simulink subsystem "Out_of_Plane_Model"  (R2025b)
settings: Solver=VariableStepAuto  StartTime=0.0  StopTime=10.0  RelTol=1e-3
undefined symbols (not defined in the file): AeroLiftCff, AeroLongDrgCff, AeroMotoEffctArea, AeroPitchMomentCff, AeroPitchMomentLngth, AeroRltWindAngVect, AeroSideFrcCff, AeroYawMomentCff, aMode, BrkFrntBrkActrBore, BrkFrntBrkActrPrsBpt, BrkFrntBrkPadMeanRadius, BrkFrntBrkTrqTbl, BrkFrntIntrnRadius, BrkFrntKinFricCff, BrkFrntPadNum, BrkFrntShoePinToDrumCntrDst, BrkFrntShoePinToFrcAppDst, BrkFrntShoePinToPadEndAng, BrkFrntShoePinToPadStartAng, BrkFrntStcFricCff, BrkFrntWhlSpdBpt, BrkRearBrkActrBore, BrkRearBrkActrPrsBpt, BrkRearBrkPadMeanRadius, BrkRearBrkTrqTbl, BrkRearIntrnRadius, BrkRearKinFricCff, BrkRearPadNum, BrkRearShoePinToDrumCntrDst, BrkRearShoePinToFrcAppDst, BrkRearShoePinToPadEndAng, BrkRearShoePinToPadStartAng, BrkRearStcFricCff, BrkRearWhlSpdBpt, CpRrVx0, CpRrVy0, CpRrY0, EnvAbsPrs, EnvAirTemp, FrkFrL0, FrmAng0, g, GasCnst, InitFrkLngth, InitMainFrmPitchAng, InitRearArmPitchAng, InitRearCntctPtchLatVel, InitRearCntctPtchLongVel, InitRearCntctPtchZ, InitYawAng, MotoFrmLngth, MotoFrmMass, MotoGrvty, MotoLatOfst, MotoLongOfst, MotoLowrFrntFrkMass, MotoPtchOfst, MotoRearArmLngth, MotoRearArmMass ... (+28)
libraries: sm_lib x309, nesl_utility_internal x158, nesl_utility x7, autolibsharedcoupling x6, vehdynlibtire x6, sharedtransform x4, shared6dof x1, matrix_library x1, vehdynlibeomcommon x1
(part 9 of 10)

== system Out_of_Plane_Model/Chassis, Tires, and Areo/Chassis Body, Suspension, and Steering/Signal routine/Ancillary_sub/Velocities/Sensor/Sensor_FrkLw ==
  PS-Simulink Converter1 : nesl_utility_internal/PS-Simulink Converter  PhysicalDomain=network_engine_domain  SubClassName=ps_output  LeftPortType=input  RightPortType=output  PseudoPeriodic=off  Frequencies=[]  VectorFormat=1-D array  Unit=inherit  AffineConversion=off
  PS-Simulink Converter4 : nesl_utility_internal/PS-Simulink Converter  PhysicalDomain=network_engine_domain  SubClassName=ps_output  LeftPortType=input  RightPortType=output  PseudoPeriodic=off  Frequencies=[]  VectorFormat=1-D array  Unit=inherit  AffineConversion=off
  PS-Simulink Converter5 : nesl_utility_internal/PS-Simulink Converter  PhysicalDomain=network_engine_domain  SubClassName=ps_output  LeftPortType=input  RightPortType=output  PseudoPeriodic=off  Frequencies=[]  VectorFormat=1-D array  Unit=inherit  AffineConversion=off
  Transform Sensor1 : sm_lib/Frames and Transforms/Transform Sensor  MeasurementFrame=NonRotatingFollower  RotationSequence=XYX  SenseAngle=off  SenseAxis=off  SenseQ=off  SenseR=off  SenseRotationSequence=off  SenseOmegaX=off  SenseOmegaY=off  SenseOmegaZ=off  SenseOmega=off  SenseQDot=off  SenseRDot=off  SenseRotationSequenceDot=off  SenseAlphaX=off  SenseAlphaY=off  SenseAlphaZ=off  SenseAlpha=off  SenseQDDot=off  SenseRDDot=off  SenseX=off  SenseY=off  SenseZ=off  SenseXYZ=off  SenseRad=off  SenseAzim=off  SenseDist=off  SenseInc=off  SenseXDot=on  SenseYDot=on  SenseZDot=on  SenseXYZDot=off  SenseRadDot=off  SenseAzimDot=off  SenseDistDot=off  SenseIncDot=off  SenseXDDot=off  SenseYDDot=off  SenseZDDot=off  SenseXYZDDot=off  SenseRadDDot=off  SenseAzimDDot=off  SenseDistDDot=off  SenseIncDDot=off
  World Frame : sm_lib/Frames and Transforms/World Frame
  F : PMIOPort  Side=Left
  Vx_vf : Outport
  Vy_vf : Outport  Port=2
  Vz_vf : Outport  Port=3
  wires:
  PS-Simulink Converter5/1 -> Vy_vf/1
  PS-Simulink Converter4/1 -> Vx_vf/1
  PS-Simulink Converter1/1 -> Vz_vf/1
  connections:
  World Frame/RConn1 -- Transform Sensor1/LConn1
  Transform Sensor1/RConn1 -- F/RConn1
  PS-Simulink Converter5/LConn1 -- Transform Sensor1/RConn3
  PS-Simulink Converter4/LConn1 -- Transform Sensor1/RConn2
  PS-Simulink Converter1/LConn1 -- Transform Sensor1/RConn4

== system Out_of_Plane_Model/Chassis, Tires, and Areo/Chassis Body, Suspension, and Steering/Signal routine/Ancillary_sub/Velocities/Sensor/Sensor_FrkUp ==
  PS-Simulink Converter1 : nesl_utility_internal/PS-Simulink Converter  PhysicalDomain=network_engine_domain  SubClassName=ps_output  LeftPortType=input  RightPortType=output  PseudoPeriodic=off  Frequencies=[]  VectorFormat=1-D array  Unit=inherit  AffineConversion=off
  PS-Simulink Converter4 : nesl_utility_internal/PS-Simulink Converter  PhysicalDomain=network_engine_domain  SubClassName=ps_output  LeftPortType=input  RightPortType=output  PseudoPeriodic=off  Frequencies=[]  VectorFormat=1-D array  Unit=inherit  AffineConversion=off
  PS-Simulink Converter5 : nesl_utility_internal/PS-Simulink Converter  PhysicalDomain=network_engine_domain  SubClassName=ps_output  LeftPortType=input  RightPortType=output  PseudoPeriodic=off  Frequencies=[]  VectorFormat=1-D array  Unit=inherit  AffineConversion=off
  Transform Sensor1 : sm_lib/Frames and Transforms/Transform Sensor  MeasurementFrame=NonRotatingFollower  RotationSequence=XYX  SenseAngle=off  SenseAxis=off  SenseQ=off  SenseR=off  SenseRotationSequence=off  SenseOmegaX=off  SenseOmegaY=off  SenseOmegaZ=off  SenseOmega=off  SenseQDot=off  SenseRDot=off  SenseRotationSequenceDot=off  SenseAlphaX=off  SenseAlphaY=off  SenseAlphaZ=off  SenseAlpha=off  SenseQDDot=off  SenseRDDot=off  SenseX=off  SenseY=off  SenseZ=off  SenseXYZ=off  SenseRad=off  SenseAzim=off  SenseDist=off  SenseInc=off  SenseXDot=on  SenseYDot=on  SenseZDot=on  SenseXYZDot=off  SenseRadDot=off  SenseAzimDot=off  SenseDistDot=off  SenseIncDot=off  SenseXDDot=off  SenseYDDot=off  SenseZDDot=off  SenseXYZDDot=off  SenseRadDDot=off  SenseAzimDDot=off  SenseDistDDot=off  SenseIncDDot=off
  World Frame : sm_lib/Frames and Transforms/World Frame
  F : PMIOPort  Side=Left
  Vx_vf : Outport
  Vy_vf : Outport  Port=2
  Vz_vf : Outport  Port=3
  wires:
  PS-Simulink Converter1/1 -> Vz_vf/1
  PS-Simulink Converter4/1 -> Vx_vf/1
  PS-Simulink Converter5/1 -> Vy_vf/1
  connections:
  PS-Simulink Converter1/LConn1 -- Transform Sensor1/RConn4
  PS-Simulink Converter4/LConn1 -- Transform Sensor1/RConn2
  PS-Simulink Converter5/LConn1 -- Transform Sensor1/RConn3
  Transform Sensor1/RConn1 -- F/RConn1
  World Frame/RConn1 -- Transform Sensor1/LConn1

== system Out_of_Plane_Model/Chassis, Tires, and Areo/Chassis Body, Suspension, and Steering/Signal routine/Ancillary_sub/Velocities/Sensor/Sensor_Frm ==
  PS-Simulink Converter1 : nesl_utility_internal/PS-Simulink Converter  PhysicalDomain=network_engine_domain  SubClassName=ps_output  LeftPortType=input  RightPortType=output  PseudoPeriodic=off  Frequencies=[]  VectorFormat=1-D array  Unit=inherit  AffineConversion=off
  PS-Simulink Converter4 : nesl_utility_internal/PS-Simulink Converter  PhysicalDomain=network_engine_domain  SubClassName=ps_output  LeftPortType=input  RightPortType=output  PseudoPeriodic=off  Frequencies=[]  VectorFormat=1-D array  Unit=inherit  AffineConversion=off
  PS-Simulink Converter5 : nesl_utility_internal/PS-Simulink Converter  PhysicalDomain=network_engine_domain  SubClassName=ps_output  LeftPortType=input  RightPortType=output  PseudoPeriodic=off  Frequencies=[]  VectorFormat=1-D array  Unit=inherit  AffineConversion=off
  Transform Sensor1 : sm_lib/Frames and Transforms/Transform Sensor  MeasurementFrame=NonRotatingFollower  RotationSequence=XYX  SenseAngle=off  SenseAxis=off  SenseQ=off  SenseR=off  SenseRotationSequence=off  SenseOmegaX=off  SenseOmegaY=off  SenseOmegaZ=off  SenseOmega=off  SenseQDot=off  SenseRDot=off  SenseRotationSequenceDot=off  SenseAlphaX=off  SenseAlphaY=off  SenseAlphaZ=off  SenseAlpha=off  SenseQDDot=off  SenseRDDot=off  SenseX=off  SenseY=off  SenseZ=off  SenseXYZ=off  SenseRad=off  SenseAzim=off  SenseDist=off  SenseInc=off  SenseXDot=on  SenseYDot=on  SenseZDot=on  SenseXYZDot=off  SenseRadDot=off  SenseAzimDot=off  SenseDistDot=off  SenseIncDot=off  SenseXDDot=off  SenseYDDot=off  SenseZDDot=off  SenseXYZDDot=off  SenseRadDDot=off  SenseAzimDDot=off  SenseDistDDot=off  SenseIncDDot=off
  World Frame : sm_lib/Frames and Transforms/World Frame
  F : PMIOPort  Side=Left
  Vx_vf : Outport
  Vy_vf : Outport  Port=2
  Vz_vf : Outport  Port=3
  wires:
  PS-Simulink Converter5/1 -> Vy_vf/1
  PS-Simulink Converter4/1 -> Vx_vf/1
  PS-Simulink Converter1/1 -> Vz_vf/1
  connections:
  World Frame/RConn1 -- Transform Sensor1/LConn1
  Transform Sensor1/RConn1 -- F/RConn1
  PS-Simulink Converter5/LConn1 -- Transform Sensor1/RConn3
  PS-Simulink Converter4/LConn1 -- Transform Sensor1/RConn2
  PS-Simulink Converter1/LConn1 -- Transform Sensor1/RConn4

== system Out_of_Plane_Model/Chassis, Tires, and Areo/Chassis Body, Suspension, and Steering/Signal routine/Ancillary_sub/Velocities/Sensor/Sensor_Rdr ==
  PS-Simulink Converter1 : nesl_utility_internal/PS-Simulink Converter  PhysicalDomain=network_engine_domain  SubClassName=ps_output  LeftPortType=input  RightPortType=output  PseudoPeriodic=off  Frequencies=[]  VectorFormat=1-D array  Unit=inherit  AffineConversion=off
  PS-Simulink Converter4 : nesl_utility_internal/PS-Simulink Converter  PhysicalDomain=network_engine_domain  SubClassName=ps_output  LeftPortType=input  RightPortType=output  PseudoPeriodic=off  Frequencies=[]  VectorFormat=1-D array  Unit=inherit  AffineConversion=off
  PS-Simulink Converter5 : nesl_utility_internal/PS-Simulink Converter  PhysicalDomain=network_engine_domain  SubClassName=ps_output  LeftPortType=input  RightPortType=output  PseudoPeriodic=off  Frequencies=[]  VectorFormat=1-D array  Unit=inherit  AffineConversion=off
  Transform Sensor1 : sm_lib/Frames and Transforms/Transform Sensor  MeasurementFrame=NonRotatingFollower  RotationSequence=XYX  SenseAngle=off  SenseAxis=off  SenseQ=off  SenseR=off  SenseRotationSequence=off  SenseOmegaX=off  SenseOmegaY=off  SenseOmegaZ=off  SenseOmega=off  SenseQDot=off  SenseRDot=off  SenseRotationSequenceDot=off  SenseAlphaX=off  SenseAlphaY=off  SenseAlphaZ=off  SenseAlpha=off  SenseQDDot=off  SenseRDDot=off  SenseX=off  SenseY=off  SenseZ=off  SenseXYZ=off  SenseRad=off  SenseAzim=off  SenseDist=off  SenseInc=off  SenseXDot=on  SenseYDot=on  SenseZDot=on  SenseXYZDot=off  SenseRadDot=off  SenseAzimDot=off  SenseDistDot=off  SenseIncDot=off  SenseXDDot=off  SenseYDDot=off  SenseZDDot=off  SenseXYZDDot=off  SenseRadDDot=off  SenseAzimDDot=off  SenseDistDDot=off  SenseIncDDot=off
  World Frame : sm_lib/Frames and Transforms/World Frame
  F : PMIOPort  Side=Left
  Vx_vf : Outport
  Vy_vf : Outport  Port=2
  Vz_vf : Outport  Port=3
  wires:
  PS-Simulink Converter5/1 -> Vy_vf/1
  PS-Simulink Converter4/1 -> Vx_vf/1
  PS-Simulink Converter1/1 -> Vz_vf/1
  connections:
  World Frame/RConn1 -- Transform Sensor1/LConn1
  Transform Sensor1/RConn1 -- F/RConn1
  PS-Simulink Converter5/LConn1 -- Transform Sensor1/RConn3
  PS-Simulink Converter4/LConn1 -- Transform Sensor1/RConn2
  PS-Simulink Converter1/LConn1 -- Transform Sensor1/RConn4

== system Out_of_Plane_Model/Chassis, Tires, and Areo/Chassis Body, Suspension, and Steering/Signal routine/Ancillary_sub/Velocities/Sensor/Sensor_WhlFr ==
  PS-Simulink Converter1 : nesl_utility_internal/PS-Simulink Converter  PhysicalDomain=network_engine_domain  SubClassName=ps_output  LeftPortType=input  RightPortType=output  PseudoPeriodic=off  Frequencies=[]  VectorFormat=1-D array  Unit=inherit  AffineConversion=off
  PS-Simulink Converter4 : nesl_utility_internal/PS-Simulink Converter  PhysicalDomain=network_engine_domain  SubClassName=ps_output  LeftPortType=input  RightPortType=output  PseudoPeriodic=off  Frequencies=[]  VectorFormat=1-D array  Unit=inherit  AffineConversion=off
  PS-Simulink Converter5 : nesl_utility_internal/PS-Simulink Converter  PhysicalDomain=network_engine_domain  SubClassName=ps_output  LeftPortType=input  RightPortType=output  PseudoPeriodic=off  Frequencies=[]  VectorFormat=1-D array  Unit=inherit  AffineConversion=off
  Transform Sensor1 : sm_lib/Frames and Transforms/Transform Sensor  MeasurementFrame=NonRotatingFollower  RotationSequence=XYX  SenseAngle=off  SenseAxis=off  SenseQ=off  SenseR=off  SenseRotationSequence=off  SenseOmegaX=off  SenseOmegaY=off  SenseOmegaZ=off  SenseOmega=off  SenseQDot=off  SenseRDot=off  SenseRotationSequenceDot=off  SenseAlphaX=off  SenseAlphaY=off  SenseAlphaZ=off  SenseAlpha=off  SenseQDDot=off  SenseRDDot=off  SenseX=off  SenseY=off  SenseZ=off  SenseXYZ=off  SenseRad=off  SenseAzim=off  SenseDist=off  SenseInc=off  SenseXDot=on  SenseYDot=on  SenseZDot=on  SenseXYZDot=off  SenseRadDot=off  SenseAzimDot=off  SenseDistDot=off  SenseIncDot=off  SenseXDDot=off  SenseYDDot=off  SenseZDDot=off  SenseXYZDDot=off  SenseRadDDot=off  SenseAzimDDot=off  SenseDistDDot=off  SenseIncDDot=off
  World Frame : sm_lib/Frames and Transforms/World Frame
  F : PMIOPort  Side=Left
  Vx_vf : Outport
  Vy_vf : Outport  Port=2
  Vz_vf : Outport  Port=3
  wires:
  PS-Simulink Converter5/1 -> Vy_vf/1
  PS-Simulink Converter4/1 -> Vx_vf/1
  PS-Simulink Converter1/1 -> Vz_vf/1
  connections:
  World Frame/RConn1 -- Transform Sensor1/LConn1
  Transform Sensor1/RConn1 -- F/RConn1
  PS-Simulink Converter5/LConn1 -- Transform Sensor1/RConn3
  PS-Simulink Converter4/LConn1 -- Transform Sensor1/RConn2
  PS-Simulink Converter1/LConn1 -- Transform Sensor1/RConn4

== system Out_of_Plane_Model/Chassis, Tires, and Areo/Chassis Body, Suspension, and Steering/Signal routine/Ancillary_sub/Velocities/Sensor/Sensor_WhlRr ==
  PS-Simulink Converter1 : nesl_utility_internal/PS-Simulink Converter  PhysicalDomain=network_engine_domain  SubClassName=ps_output  LeftPortType=input  RightPortType=output  PseudoPeriodic=off  Frequencies=[]  VectorFormat=1-D array  Unit=inherit  AffineConversion=off
  PS-Simulink Converter4 : nesl_utility_internal/PS-Simulink Converter  PhysicalDomain=network_engine_domain  SubClassName=ps_output  LeftPortType=input  RightPortType=output  PseudoPeriodic=off  Frequencies=[]  VectorFormat=1-D array  Unit=inherit  AffineConversion=off
  PS-Simulink Converter5 : nesl_utility_internal/PS-Simulink Converter  PhysicalDomain=network_engine_domain  SubClassName=ps_output  LeftPortType=input  RightPortType=output  PseudoPeriodic=off  Frequencies=[]  VectorFormat=1-D array  Unit=inherit  AffineConversion=off
  Transform Sensor1 : sm_lib/Frames and Transforms/Transform Sensor  MeasurementFrame=NonRotatingFollower  RotationSequence=XYX  SenseAngle=off  SenseAxis=off  SenseQ=off  SenseR=off  SenseRotationSequence=off  SenseOmegaX=off  SenseOmegaY=off  SenseOmegaZ=off  SenseOmega=off  SenseQDot=off  SenseRDot=off  SenseRotationSequenceDot=off  SenseAlphaX=off  SenseAlphaY=off  SenseAlphaZ=off  SenseAlpha=off  SenseQDDot=off  SenseRDDot=off  SenseX=off  SenseY=off  SenseZ=off  SenseXYZ=off  SenseRad=off  SenseAzim=off  SenseDist=off  SenseInc=off  SenseXDot=on  SenseYDot=on  SenseZDot=on  SenseXYZDot=off  SenseRadDot=off  SenseAzimDot=off  SenseDistDot=off  SenseIncDot=off  SenseXDDot=off  SenseYDDot=off  SenseZDDot=off  SenseXYZDDot=off  SenseRadDDot=off  SenseAzimDDot=off  SenseDistDDot=off  SenseIncDDot=off
  World Frame : sm_lib/Frames and Transforms/World Frame
  F : PMIOPort  Side=Left
  Vx_vf : Outport
  Vy_vf : Outport  Port=2
  Vz_vf : Outport  Port=3
  wires:
  PS-Simulink Converter1/1 -> Vz_vf/1
  PS-Simulink Converter4/1 -> Vx_vf/1
  PS-Simulink Converter5/1 -> Vy_vf/1
  connections:
  PS-Simulink Converter1/LConn1 -- Transform Sensor1/RConn4
  PS-Simulink Converter4/LConn1 -- Transform Sensor1/RConn2
  PS-Simulink Converter5/LConn1 -- Transform Sensor1/RConn3
  Transform Sensor1/RConn1 -- F/RConn1
  World Frame/RConn1 -- Transform Sensor1/LConn1

== system Out_of_Plane_Model/Chassis, Tires, and Areo/Chassis Body, Suspension, and Steering/Signal routine/Info_sub/BdyFrm/CG/centripetal ==
  p : Inport
  q : Inport  Port=2
  r : Inport  Port=3
  xdot : Inport  Port=4
  ydot : Inport  Port=5
  zdot : Inport  Port=6
  xddot : Inport  Port=7
  yddot : Inport  Port=8
  zddot : Inport  Port=9
  Add : Sum
  Cross Product : matrix_library/Cross Product
  Demux4 : Demux  Outputs=3
  Mux : Mux  Inputs=3
  Mux1 : Mux  Inputs=3
  Mux2 : Mux  Inputs=3
  ax : Outport
  ay : Outport  Port=2
  az : Outport  Port=3
  wires:
  Mux/1 -> Cross Product/1
  Demux4/1 -> ax/1
  Mux1/1 -> Cross Product/2
  Cross Product/1 -> Add/1
  Mux2/1 -> Add/2
  zdot/1 -> Mux1/3
  p/1 -> Mux/1
  Add/1 -> Demux4/1
  q/1 -> Mux/2
  yddot/1 -> Mux2/2
  Demux4/2 -> ay/1
  r/1 -> Mux/3
  Demux4/3 -> az/1
  ydot/1 -> Mux1/2
  xdot/1 -> Mux1/1
  zddot/1 -> Mux2/3
  xddot/1 -> Mux2/1

== system Out_of_Plane_Model/Chassis, Tires, and Areo/Tire/Front Tire/Linear Front Simscape Tire/Brake model/MW Brake/Brakes ==
  note: 1) Add Subsystem or Model blocks as valid variant choices.
      | 2) You cannot connect blocks at this level. At simulation, connectivity is automatically
      | determined, based on the active variant and port name matching.
  BrkPrs : Inport
  Omega : Inport  Port=2
  Disk Brake : Subsystem  VariantControl=Disk
  Drum Brake : Subsystem  VariantControl=Drum
  Mapped Brake : Subsystem  VariantControl=Mapped
  No Brake : Subsystem  VariantControl=None
  MyBrk : Outport  VectorParamsAs1DForOutWhenUnconnected=off

== system Out_of_Plane_Model/Chassis, Tires, and Areo/Tire/Front Tire/Linear Front Simscape Tire/Contact model/Simple spring and damper/contact decision ==
  pos : Inport
  Fpre : Inport  Port=2
  Add2 : Sum
  Constant1 : Constant  Value=0.5
  Divide1 : Product  Inputs=**
  Gain12 : Gain  Gain=0.5
  Sign1 : Signum  ZeroCross=off
  F : Outport  VectorParamsAs1DForOutWhenUnconnected=off
  wires:
  Gain12/1 -> Add2/1
  pos/1 -> Sign1/1
  Constant1/1 -> Add2/2
  Sign1/1 -> Gain12/1
  Add2/1 -> Divide1/1
  Fpre/1 -> Divide1/2
  Divide1/1 -> F/1

== system Out_of_Plane_Model/Chassis, Tires, and Areo/Tire/Front Tire/Linear Front Simscape Tire/Friction model/External/Calc. part Vertical load & SideSlipAngle ==
  vel. : Inport
  Atan2 : Trigonometry  Operator=atan2
  Demux : Demux  Outputs=3
  Divide1 : Product  Inputs=**
  Gain : Gain  Gain=-1
  Pythagorean theorem : Subsystem
  Sign : Signum  ZeroCross=off
  Terminator : Terminator
  Road Vel. : Outport  VectorParamsAs1DForOutWhenUnconnected=off
  SideSlipAngle [rad] : Outport  Port=2  VectorParamsAs1DForOutWhenUnconnected=off
  wires:
  Demux/2 -> Pythagorean theorem/2(Y), Gain/1  "Vy"
  Demux/3 -> Terminator/1  "Vz"
  vel./1 -> Demux/1
  Demux/1 -> Atan2/2, Sign/1, Pythagorean theorem/1(X)
  Atan2/1 -> SideSlipAngle [rad]/1
  Gain/1 -> Atan2/1
  Pythagorean theorem/1(sqrt(X^2+Y^2)) -> Divide1/2
  Sign/1 -> Divide1/1
  Divide1/1 -> Road Vel./1

== system Out_of_Plane_Model/Chassis, Tires, and Areo/Tire/Front Tire/Linear Front Simscape Tire/Friction model/External/SlipRatio ==
  RoadVelocity : Inport
  Rot.Velocity : Inport  Port=2
  Slip : vehdynlibtire/Dugoff Wheel 2DOF/Dugoff/Slip  mask{Lrelx=.15, KPUMAX=0.95, KPUMIN=-0.95}
      mask prompts: Lrelx "Relaxation length [m]:"; KPUMAX "Maximum slip ratio [-]:"; KPUMIN "Minimum slip ratio [-]:"
      settings: LibrarySourceBlock=vehdynlibtire/Fiala Wheel 2DOF/Fiala/Slip
  Tire radius : Constant  Value=RWhl
  Unary Minus : UnaryMinus
  SlipRatio : Outport  VectorParamsAs1DForOutWhenUnconnected=off
  wires:
  RoadVelocity/1 -> Slip/2
  Rot.Velocity/1 -> Unary Minus/1
  Slip/1 -> SlipRatio/1
  Tire radius/1 -> Slip/3
  Unary Minus/1 -> Slip/1

== system Out_of_Plane_Model/Chassis, Tires, and Areo/Tire/Front Tire/Linear Front Simscape Tire/Friction model/Linear/SlipRatio ==
  RoadVelocity : Inport
  Rot.Velocity : Inport  Port=2
  Slip : vehdynlibtire/Dugoff Wheel 2DOF/Dugoff/Slip  mask{Lrelx=0.15, KPUMAX=0.95, KPUMIN=-0.95}
      mask prompts: Lrelx "Relaxation length [m]:"; KPUMAX "Maximum slip ratio [-]:"; KPUMIN "Minimum slip ratio [-]:"
      settings: LibrarySourceBlock=vehdynlibtire/Fiala Wheel 2DOF/Fiala/Slip
  Tire radius : Constant  Value=RWhl
  Unary Minus : UnaryMinus
  Unary Minus1 : UnaryMinus
  SlipRatio : Outport  VectorParamsAs1DForOutWhenUnconnected=off
  wires:
  Unary Minus/1 -> Slip/1
  Rot.Velocity/1 -> Unary Minus/1
  RoadVelocity/1 -> Slip/2
  Tire radius/1 -> Slip/3
  Slip/1 -> Unary Minus1/1
  Unary Minus1/1 -> SlipRatio/1

== system Out_of_Plane_Model/Chassis, Tires, and Areo/Tire/Front Tire/Linear Front Simscape Tire/Friction model/LinearOld/Calc. part Vertical load & SideSlipAngle ==
  vel. : Inport
  Add : Sum
  Constant : Constant  Value=1e-5
  Demux : Demux  Outputs=3
  Divide : Product  Inputs=*/
  Gain : Gain  Gain=-1
  Pythagorean theorem : Subsystem
  Terminator : Terminator
  Trigonometric Function : Trigonometry  Operator=atan
  Road Vel. : Outport  VectorParamsAs1DForOutWhenUnconnected=off
  SideSlipAngle [rad] : Outport  Port=2  VectorParamsAs1DForOutWhenUnconnected=off
  wires:
  Gain/1 -> Divide/1
  Demux/2 -> Pythagorean theorem/2(Y), Gain/1  "Vy"
  Demux/3 -> Terminator/1  "Vz"
  Trigonometric Function/1 -> SideSlipAngle [rad]/1
  vel./1 -> Demux/1
  Pythagorean theorem/1(sqrt(X^2+Y^2)) -> Road Vel./1
  Divide/1 -> Trigonometric Function/1
  Demux/1 -> Add/1, Pythagorean theorem/1(X)  "Vx"
  Add/1 -> Divide/2
  Constant/1 -> Add/2

== system Out_of_Plane_Model/Chassis, Tires, and Areo/Tire/Front Tire/Linear Front Simscape Tire/Friction model/LinearOld/SlipRatio ==
  RoadVelocity : Inport
  SlipAngle : Inport  Port=2
  Rot.Velocity : Inport  Port=3
  Abs : Abs  ZeroCross=off  SaturateOnIntegerOverflow=off
  Constant : Constant  Value=-0.95
  Sign : Signum  ZeroCross=off
  Slip Ratio _ Braking : Subsystem
  Slip Ratio _ Driving : Subsystem
  Switch : Switch  Criteria=u2 > Threshold  ZeroCross=off  SaturateOnIntegerOverflow=off  InputSameDT=off
  Switch1 : Switch  Threshold=1  ZeroCross=off  SaturateOnIntegerOverflow=off  InputSameDT=off
  Switch2 : Switch  Threshold=-0.95  ZeroCross=off  SaturateOnIntegerOverflow=off  InputSameDT=off
  Unary Minus : UnaryMinus
  SlipRatio : Outport  VectorParamsAs1DForOutWhenUnconnected=off
  wires:
  RoadVelocity/1 -> Slip Ratio _ Braking/1(RoadVelocity), Slip Ratio _ Driving/1(Road velocity)
  SlipAngle/1 -> Slip Ratio _ Braking/2(SlipAngle), Slip Ratio _ Driving/2(SlipAngle)
  Slip Ratio _ Braking/2(Switch flag) -> Switch/2
  Slip Ratio _ Driving/1(Sbd) -> Switch/3
  Rot.Velocity/1 -> Unary Minus/1
  Slip Ratio _ Braking/1(Sbb) -> Switch/1
  Switch/1 -> Switch1/3, Sign/1, Abs/1
  Abs/1 -> Switch1/2
  Sign/1 -> Switch1/1
  Constant/1 -> Switch2/3
  Switch1/1 -> Switch2/1, Switch2/2
  Unary Minus/1 -> Slip Ratio _ Braking/3(Rot.Velocity), Slip Ratio _ Driving/3(Rot.Velocity)
  Switch2/1 -> SlipRatio/1

== system Out_of_Plane_Model/Chassis, Tires, and Areo/Tire/Front Tire/Linear Front Simscape Tire/Simscape/Simscape Multibody Rim&Wheel/Tire_Rim_wth_transient ==
  Ext.F_T : Inport
  " Frame_CP" : sm_lib/Body Elements/Graphic  GraphicType=Marker  MarkerShape=Frame  MarkerSize=100  GraphicVisPropType=SimpleVisualProperties  GraphicDiffuseColor=[0.6 0.6 0.0]  GraphicOpacity=1.0  GraphicSpecularColor=[0.5 0.5 0.5 1.0]  GraphicAmbientColor=[0.15 0.15 0.15 1.0]  GraphicEmissiveColor=[0.0 0.0 0.0 1.0]  GraphicShininess=75
  Angle Constraint : sm_lib/Constraints/Angle Constraint  ConstraintType=Parallel  Angle=pi  AngleUnits=rad  WrenchDir=FollowerOnBase  WrenchFrame=BaseFrame  SenseTorque=off  SenseSignedTorqueMagnitude=off
  Bus Creator : BusCreator  Inputs=4
  CPSensor : Subsystem
  Cylindrical Solid : sm_lib/Body Elements/Cylindrical Solid  CylinderRadius=RWhl  CylinderRadiusUnits=m  CylinderLength=0.12  CylinderLengthUnits=m  ExportEntireGeometry=off  InertiaType=Custom  BasedOnType=Density  Density=1000  DensityUnits=kg/m^3  Mass=WhlMass  MassUnits=kg  CenterOfMass=[0 0 0]  CenterOfMassUnits=m  MomentsOfInertia=[whlInert(1), whlInert(3), whlInert(2)]  MomentsOfInertiaUnits=kg*m^2  ProductsOfInertia=[0 0 0]  ProductsOfInertiaUnits=kg*m^2  GraphicType=FromGeometry  MarkerShape=Sphere  MarkerSize=10  GraphicVisPropType=SimpleVisualProperties  GraphicDiffuseColor=[0.4 0.4 1.0]  GraphicOpacity=1  GraphicSpecularColor=[0.5 0.5 0.5 1.0]  GraphicAmbientColor=[0.15 0.15 0.15 1.0]  GraphicEmissiveColor=[0.0 0.0 0.0 1.0]  GraphicShininess=75  DoExposeReferenceFrame=on  SerializedFrames=<Frames/>
  Dummy mass : sm_lib/Body Elements/Brick Solid  BrickDimensions=[1 1 1]*1e-3  BrickDimensionsUnits=m  ExportEntireGeometry=off  InertiaType=Custom  BasedOnType=Density  Density=1000  DensityUnits=kg/m^3  Mass=1e-6  MassUnits=kg  CenterOfMass=[0 0 0]  CenterOfMassUnits=m  MomentsOfInertia=[1 1 1]*1e-10  MomentsOfInertiaUnits=kg*m^2  ProductsOfInertia=[0 0 0]  ProductsOfInertiaUnits=kg*m^2  GraphicType=FromGeometry  MarkerShape=Sphere  MarkerSize=10  GraphicVisPropType=SimpleVisualProperties  GraphicDiffuseColor=[0.5 0.5 0.5]  GraphicOpacity=1.0  GraphicSpecularColor=[0.5 0.5 0.5 1.0]  GraphicAmbientColor=[0.15 0.15 0.15 1.0]  GraphicEmissiveColor=[0.0 0.0 0.0 1.0]  GraphicShininess=75  DoExposeReferenceFrame=on  SerializedFrames=<Frames/>
  External Force and Torque : sm_lib/Forces and Torques/External Force and Torque  EnableForceX=off  EnableForceY=off  EnableForceZ=off  EnableForce=off  ForceResolutionFrame=World  EnableTorqueX=off  EnableTorqueY=on  EnableTorqueZ=off  EnableTorque=off  TorqueResolutionFrame=AttachedFrame
  Graphic : sm_lib/Body Elements/Graphic  GraphicType=Marker  MarkerShape=Frame  MarkerSize=20  GraphicVisPropType=SimpleVisualProperties  GraphicDiffuseColor=[1.0 1.0 1.0]  GraphicOpacity=1.0  GraphicSpecularColor=[0.5 0.5 0.5 1.0]  GraphicAmbientColor=[0.15 0.15 0.15 1.0]  GraphicEmissiveColor=[0.0 0.0 0.0 1.0]  GraphicShininess=75
  Pitch dof : Subsystem
  Rigid Transform1 : sm_lib/Frames and Transforms/Rigid Transform  RotationMethod=None  FollAlignAxisA=+X  BaseAlignAxisA=+Y  FollAlignAxisB=+Y  BaseAlignAxisB=+Z  RotationStandardAxis=+X  RotationAngle=0  RotationAngleUnits=rad  RotationArbitraryAxis=[0 0 1]  RotationSequenceAxes=FollowerAxes  RotationSequence=XYX  RotationSequenceAngles=[0 0 0]  RotationSequenceAnglesUnits=deg  RotationMatrix=[1 0 0; 0 1 0; 0 0 1]  Quaternion=[1 0 0 0]  TranslationMethod=Cartesian  TranslationCartesianOffset=[0 0 RWhl]  TranslationCartesianOffsetUnits=m  TranslationStandardAxis=+X  TranslationStandardOffset=0  TranslationStandardOffsetUnits=m  TranslationROffset=0  TranslationROffsetUnits=m  TranslationThetaOffset=0  TranslationThetaOffsetUnits=deg  TranslationZOffset=0  TranslationZOffsetUnits=m
  Rigid Transform2 : sm_lib/Frames and Transforms/Rigid Transform  RotationMethod=StandardAxis  FollAlignAxisA=+X  BaseAlignAxisA=+Y  FollAlignAxisB=+Y  BaseAlignAxisB=+Z  RotationStandardAxis=-X  RotationAngle=pi/2  RotationAngleUnits=rad  RotationArbitraryAxis=[0 0 1]  RotationSequenceAxes=FollowerAxes  RotationSequence=XYX  RotationSequenceAngles=[0 0 0]  RotationSequenceAnglesUnits=deg  RotationMatrix=[1 0 0; 0 1 0; 0 0 1]  Quaternion=[1 0 0 0]  TranslationMethod=None  TranslationCartesianOffset=[0 0 0]  TranslationCartesianOffsetUnits=m  TranslationStandardAxis=+X  TranslationStandardOffset=0  TranslationStandardOffsetUnits=m  TranslationROffset=0  TranslationROffsetUnits=m  TranslationThetaOffset=0  TranslationThetaOffsetUnits=deg  TranslationZOffset=0  TranslationZOffsetUnits=m
  Rigid Transform3 : sm_lib/Frames and Transforms/Rigid Transform  RotationMethod=StandardAxis  FollAlignAxisA=+X  BaseAlignAxisA=+Y  FollAlignAxisB=+Y  BaseAlignAxisB=+Z  RotationStandardAxis=+X  RotationAngle=pi  RotationAngleUnits=rad  RotationArbitraryAxis=[0 0 1]  RotationSequenceAxes=FollowerAxes  RotationSequence=XYX  RotationSequenceAngles=[0 0 0]  RotationSequenceAnglesUnits=deg  RotationMatrix=[1 0 0; 0 1 0; 0 0 1]  Quaternion=[1 0 0 0]  TranslationMethod=None  TranslationCartesianOffset=[0 0 0]  TranslationCartesianOffsetUnits=m  TranslationStandardAxis=+X  TranslationStandardOffset=0  TranslationStandardOffsetUnits=m  TranslationROffset=0  TranslationROffsetUnits=m  TranslationThetaOffset=0  TranslationThetaOffsetUnits=deg  TranslationZOffset=0  TranslationZOffsetUnits=m
  Roll dof : Subsystem
  Simulink-PS Converter1 : nesl_utility_internal/Simulink-PS Converter  PhysicalDomain=network_engine_domain  SubClassName=ps_input  LeftPortType=input  RightPortType=output  PseudoPeriodic=off  Frequencies=[]  NoiseDistribution=none  NoiseParameters=[]  Unit=1  AffineConversion=off  FilteringAndDerivatives=provide  SimscapeFilterOrder=1  InputFilterTimeConstant=0.001  UdotUserProvided=0
  World Frame : sm_lib/Frames and Transforms/World Frame
  dofPitch : Subsystem
  Hub : PMIOPort  Side=Left
  CP : PMIOPort  Port=2  Side=Left
  omega : Outport
  omegadot : Outport  Port=2
  A,V,P_WhlRoll : Outport  Port=3
  Info_CP : Outport  Port=4
  wires:
  Bus Creator/1 -> Info_CP/1
  CPSensor/3(WhlCpZ) -> Bus Creator/3
  CPSensor/2(WhlCpY) -> Bus Creator/2
  CPSensor/1(WhlCpX) -> Bus Creator/1
  Roll dof/1(A,V,P_WhlRoll) -> A,V,P_WhlRoll/1
  Ext.F_T/1 -> Simulink-PS Converter1/1
  dofPitch/1(omega) -> omega/1  "omega"
  CPSensor/4(WhlCpVPsi) -> Bus Creator/4
  dofPitch/2(omegadot) -> omegadot/1
  connections:
  Simulink-PS Converter1/RConn1 -- External Force and Torque/LConn1
  External Force and Torque/RConn1 -- Rigid Transform2/LConn1 -- dofPitch/RConn1
  Cylindrical Solid/RConn1 -- Graphic/RConn1 -- Rigid Transform2/RConn1
  Pitch dof/LConn1 -- Hub/RConn1
  " Frame_CP"/RConn1 -- Roll dof/RConn1 -- Dummy mass/RConn1 -- CPSensor/RConn1 -- CP/RConn1 -- Angle Constraint/LConn1
  Rigid Transform1/RConn1 -- Roll dof/LConn1
  Rigid Transform3/LConn1 -- World Frame/RConn1
  Angle Constraint/RConn1 -- Rigid Transform3/RConn1
  dofPitch/LConn1 -- Rigid Transform1/LConn1 -- Pitch dof/RConn1

== system Out_of_Plane_Model/Chassis, Tires, and Areo/Tire/Rear Tire/Linear Rear Simscape Tire/Brake model/MW Brake/Brakes ==
  note: 1) Add Subsystem or Model blocks as valid variant choices.
      | 2) You cannot connect blocks at this level. At simulation, connectivity is automatically
      | determined, based on the active variant and port name matching.
  BrkPrs : Inport
  Omega : Inport  Port=2
  Disk Brake : Subsystem  VariantControl=Disk
  Drum Brake : Subsystem  VariantControl=Drum
  Mapped Brake : Subsystem  VariantControl=Mapped
  No Brake : Subsystem  VariantControl=None
  MyBrk : Outport  VectorParamsAs1DForOutWhenUnconnected=off

== system Out_of_Plane_Model/Chassis, Tires, and Areo/Tire/Rear Tire/Linear Rear Simscape Tire/Contact model/Simple spring and damper/contact decision ==
  pos : Inport
  Fpre : Inport  Port=2
  Add2 : Sum
  Constant1 : Constant  Value=0.5
  Divide1 : Product  Inputs=**
  Gain12 : Gain  Gain=0.5
  Sign1 : Signum  ZeroCross=off
  F : Outport  VectorParamsAs1DForOutWhenUnconnected=off
  wires:
  Gain12/1 -> Add2/1
  pos/1 -> Sign1/1
  Constant1/1 -> Add2/2
  Sign1/1 -> Gain12/1
  Add2/1 -> Divide1/1
  Fpre/1 -> Divide1/2
  Divide1/1 -> F/1

== system Out_of_Plane_Model/Chassis, Tires, and Areo/Tire/Rear Tire/Linear Rear Simscape Tire/Friction model/External/Calc. part Vertical load & SideSlipAngle ==
  vel. : Inport
  Atan2 : Trigonometry  Operator=atan2
  Demux : Demux  Outputs=3
  Divide1 : Product  Inputs=**
  Gain : Gain  Gain=-1
  Pythagorean theorem : Subsystem
  Sign : Signum  ZeroCross=off
  Terminator : Terminator
  Road Vel. : Outport  VectorParamsAs1DForOutWhenUnconnected=off
  SideSlipAngle [rad] : Outport  Port=2  VectorParamsAs1DForOutWhenUnconnected=off
  wires:
  Demux/2 -> Pythagorean theorem/2(Y), Gain/1  "Vy"
  Demux/3 -> Terminator/1  "Vz"
  vel./1 -> Demux/1
  Demux/1 -> Atan2/2, Sign/1, Pythagorean theorem/1(X)
  Atan2/1 -> SideSlipAngle [rad]/1
  Gain/1 -> Atan2/1
  Pythagorean theorem/1(sqrt(X^2+Y^2)) -> Divide1/2
  Sign/1 -> Divide1/1
  Divide1/1 -> Road Vel./1

== system Out_of_Plane_Model/Chassis, Tires, and Areo/Tire/Rear Tire/Linear Rear Simscape Tire/Friction model/External/SlipRatio ==
  RoadVelocity : Inport
  Rot.Velocity : Inport  Port=2
  Slip : vehdynlibtire/Dugoff Wheel 2DOF/Dugoff/Slip  mask{Lrelx=.15, KPUMAX=0.95, KPUMIN=-0.95}
      mask prompts: Lrelx "Relaxation length [m]:"; KPUMAX "Maximum slip ratio [-]:"; KPUMIN "Minimum slip ratio [-]:"
      settings: LibrarySourceBlock=vehdynlibtire/Fiala Wheel 2DOF/Fiala/Slip
  Tire radius : Constant  Value=RWhl
  Unary Minus : UnaryMinus
  SlipRatio : Outport  VectorParamsAs1DForOutWhenUnconnected=off
  wires:
  RoadVelocity/1 -> Slip/2
  Rot.Velocity/1 -> Unary Minus/1
  Slip/1 -> SlipRatio/1
  Tire radius/1 -> Slip/3
  Unary Minus/1 -> Slip/1

== system Out_of_Plane_Model/Chassis, Tires, and Areo/Tire/Rear Tire/Linear Rear Simscape Tire/Friction model/Linear/SlipRatio ==
  RoadVelocity : Inport
  Rot.Velocity : Inport  Port=2
  Slip : vehdynlibtire/Dugoff Wheel 2DOF/Dugoff/Slip  mask{Lrelx=0.15, KPUMAX=0.95, KPUMIN=-0.95}
      mask prompts: Lrelx "Relaxation length [m]:"; KPUMAX "Maximum slip ratio [-]:"; KPUMIN "Minimum slip ratio [-]:"
      settings: LibrarySourceBlock=vehdynlibtire/Fiala Wheel 2DOF/Fiala/Slip
  Tire radius : Constant  Value=RWhl
  Unary Minus : UnaryMinus
  Unary Minus1 : UnaryMinus
  SlipRatio : Outport  VectorParamsAs1DForOutWhenUnconnected=off
  wires:
  Unary Minus/1 -> Slip/1
  Rot.Velocity/1 -> Unary Minus/1
  RoadVelocity/1 -> Slip/2
  Tire radius/1 -> Slip/3
  Slip/1 -> Unary Minus1/1
  Unary Minus1/1 -> SlipRatio/1

== system Out_of_Plane_Model/Chassis, Tires, and Areo/Tire/Rear Tire/Linear Rear Simscape Tire/Friction model/LinearOld/Calc. part Vertical load & SideSlipAngle ==
  vel. : Inport
  Add : Sum
  Constant : Constant  Value=1e-5
  Demux : Demux  Outputs=3
  Divide : Product  Inputs=*/
  Gain : Gain  Gain=-1
  Pythagorean theorem : Subsystem
  Terminator : Terminator
  Trigonometric Function : Trigonometry  Operator=atan
  Road Vel. : Outport  VectorParamsAs1DForOutWhenUnconnected=off
  SideSlipAngle [rad] : Outport  Port=2  VectorParamsAs1DForOutWhenUnconnected=off
  wires:
  Gain/1 -> Divide/1
  Demux/2 -> Pythagorean theorem/2(Y), Gain/1  "Vy"
  Demux/3 -> Terminator/1  "Vz"
  Trigonometric Function/1 -> SideSlipAngle [rad]/1
  vel./1 -> Demux/1
  Pythagorean theorem/1(sqrt(X^2+Y^2)) -> Road Vel./1
  Divide/1 -> Trigonometric Function/1
  Demux/1 -> Add/1, Pythagorean theorem/1(X)  "Vx"
  Add/1 -> Divide/2
  Constant/1 -> Add/2

== system Out_of_Plane_Model/Chassis, Tires, and Areo/Tire/Rear Tire/Linear Rear Simscape Tire/Friction model/LinearOld/SlipRatio ==
  RoadVelocity : Inport
  SlipAngle : Inport  Port=2
  Rot.Velocity : Inport  Port=3
  Abs : Abs  ZeroCross=off  SaturateOnIntegerOverflow=off
  Constant : Constant  Value=-0.95
  Sign : Signum  ZeroCross=off
  Slip Ratio _ Braking : Subsystem
  Slip Ratio _ Driving : Subsystem
  Switch : Switch  Criteria=u2 > Threshold  ZeroCross=off  SaturateOnIntegerOverflow=off  InputSameDT=off
  Switch1 : Switch  Threshold=1  ZeroCross=off  SaturateOnIntegerOverflow=off  InputSameDT=off
  Switch2 : Switch  Threshold=-0.95  ZeroCross=off  SaturateOnIntegerOverflow=off  InputSameDT=off
  Unary Minus : UnaryMinus
  SlipRatio : Outport  VectorParamsAs1DForOutWhenUnconnected=off
  wires:
  RoadVelocity/1 -> Slip Ratio _ Braking/1(RoadVelocity), Slip Ratio _ Driving/1(Road velocity)
  SlipAngle/1 -> Slip Ratio _ Braking/2(SlipAngle), Slip Ratio _ Driving/2(SlipAngle)
  Slip Ratio _ Braking/2(Switch flag) -> Switch/2
  Slip Ratio _ Driving/1(Sbd) -> Switch/3
  Rot.Velocity/1 -> Unary Minus/1
  Slip Ratio _ Braking/1(Sbb) -> Switch/1
  Switch/1 -> Switch1/3, Sign/1, Abs/1
  Abs/1 -> Switch1/2
  Sign/1 -> Switch1/1
  Constant/1 -> Switch2/3
  Switch1/1 -> Switch2/1, Switch2/2
  Unary Minus/1 -> Slip Ratio _ Braking/3(Rot.Velocity), Slip Ratio _ Driving/3(Rot.Velocity)
  Switch2/1 -> SlipRatio/1

== system Out_of_Plane_Model/Chassis, Tires, and Areo/Tire/Rear Tire/Linear Rear Simscape Tire/Simscape/Simscape Multibody Rim&Wheel/Tire_Rim_wth_transient ==
  Ext.F_T : Inport
  " Frame_CP" : sm_lib/Body Elements/Graphic  GraphicType=Marker  MarkerShape=Frame  MarkerSize=100  GraphicVisPropType=SimpleVisualProperties  GraphicDiffuseColor=[0.6 0.6 0.0]  GraphicOpacity=1.0  GraphicSpecularColor=[0.5 0.5 0.5 1.0]  GraphicAmbientColor=[0.15 0.15 0.15 1.0]  GraphicEmissiveColor=[0.0 0.0 0.0 1.0]  GraphicShininess=75
  Angle Constraint : sm_lib/Constraints/Angle Constraint  ConstraintType=Parallel  Angle=pi  AngleUnits=rad  WrenchDir=FollowerOnBase  WrenchFrame=BaseFrame  SenseTorque=off  SenseSignedTorqueMagnitude=off
  Bus Creator : BusCreator  Inputs=4
  CPSensor : Subsystem
  Cylindrical Solid : sm_lib/Body Elements/Cylindrical Solid  CylinderRadius=RWhl  CylinderRadiusUnits=m  CylinderLength=0.12  CylinderLengthUnits=m  ExportEntireGeometry=off  InertiaType=Custom  BasedOnType=Density  Density=1000  DensityUnits=kg/m^3  Mass=WhlMass  MassUnits=kg  CenterOfMass=[0 0 0]  CenterOfMassUnits=m  MomentsOfInertia=[whlInert(1), whlInert(3), whlInert(2)]  MomentsOfInertiaUnits=kg*m^2  ProductsOfInertia=[0 0 0]  ProductsOfInertiaUnits=kg*m^2  GraphicType=FromGeometry  MarkerShape=Sphere  MarkerSize=10  GraphicVisPropType=SimpleVisualProperties  GraphicDiffuseColor=[0.4 0.4 1.0]  GraphicOpacity=1  GraphicSpecularColor=[0.5 0.5 0.5 1.0]  GraphicAmbientColor=[0.15 0.15 0.15 1.0]  GraphicEmissiveColor=[0.0 0.0 0.0 1.0]  GraphicShininess=75  DoExposeReferenceFrame=on  SerializedFrames=<Frames/>
  Dummy mass : sm_lib/Body Elements/Brick Solid  BrickDimensions=[1 1 1]*1e-3  BrickDimensionsUnits=m  ExportEntireGeometry=off  InertiaType=Custom  BasedOnType=Density  Density=1000  DensityUnits=kg/m^3  Mass=1e-6  MassUnits=kg  CenterOfMass=[0 0 0]  CenterOfMassUnits=m  MomentsOfInertia=[1 1 1]*1e-10  MomentsOfInertiaUnits=kg*m^2  ProductsOfInertia=[0 0 0]  ProductsOfInertiaUnits=kg*m^2  GraphicType=FromGeometry  MarkerShape=Sphere  MarkerSize=10  GraphicVisPropType=SimpleVisualProperties  GraphicDiffuseColor=[0.5 0.5 0.5]  GraphicOpacity=1.0  GraphicSpecularColor=[0.5 0.5 0.5 1.0]  GraphicAmbientColor=[0.15 0.15 0.15 1.0]  GraphicEmissiveColor=[0.0 0.0 0.0 1.0]  GraphicShininess=75  DoExposeReferenceFrame=on  SerializedFrames=<Frames/>
  External Force and Torque : sm_lib/Forces and Torques/External Force and Torque  EnableForceX=off  EnableForceY=off  EnableForceZ=off  EnableForce=off  ForceResolutionFrame=World  EnableTorqueX=off  EnableTorqueY=on  EnableTorqueZ=off  EnableTorque=off  TorqueResolutionFrame=AttachedFrame
  Graphic : sm_lib/Body Elements/Graphic  GraphicType=Marker  MarkerShape=Frame  MarkerSize=20  GraphicVisPropType=SimpleVisualProperties  GraphicDiffuseColor=[1.0 1.0 1.0]  GraphicOpacity=1.0  GraphicSpecularColor=[0.5 0.5 0.5 1.0]  GraphicAmbientColor=[0.15 0.15 0.15 1.0]  GraphicEmissiveColor=[0.0 0.0 0.0 1.0]  GraphicShininess=75
  Pitch dof : Subsystem
  Rigid Transform1 : sm_lib/Frames and Transforms/Rigid Transform  RotationMethod=None  FollAlignAxisA=+X  BaseAlignAxisA=+Y  FollAlignAxisB=+Y  BaseAlignAxisB=+Z  RotationStandardAxis=+X  RotationAngle=0  RotationAngleUnits=rad  RotationArbitraryAxis=[0 0 1]  RotationSequenceAxes=FollowerAxes  RotationSequence=XYX  RotationSequenceAngles=[0 0 0]  RotationSequenceAnglesUnits=deg  RotationMatrix=[1 0 0; 0 1 0; 0 0 1]  Quaternion=[1 0 0 0]  TranslationMethod=Cartesian  TranslationCartesianOffset=[0 0 RWhl]  TranslationCartesianOffsetUnits=m  TranslationStandardAxis=+X  TranslationStandardOffset=0  TranslationStandardOffsetUnits=m  TranslationROffset=0  TranslationROffsetUnits=m  TranslationThetaOffset=0  TranslationThetaOffsetUnits=deg  TranslationZOffset=0  TranslationZOffsetUnits=m
  Rigid Transform2 : sm_lib/Frames and Transforms/Rigid Transform  RotationMethod=StandardAxis  FollAlignAxisA=+X  BaseAlignAxisA=+Y  FollAlignAxisB=+Y  BaseAlignAxisB=+Z  RotationStandardAxis=-X  RotationAngle=pi/2  RotationAngleUnits=rad  RotationArbitraryAxis=[0 0 1]  RotationSequenceAxes=FollowerAxes  RotationSequence=XYX  RotationSequenceAngles=[0 0 0]  RotationSequenceAnglesUnits=deg  RotationMatrix=[1 0 0; 0 1 0; 0 0 1]  Quaternion=[1 0 0 0]  TranslationMethod=None  TranslationCartesianOffset=[0 0 0]  TranslationCartesianOffsetUnits=m  TranslationStandardAxis=+X  TranslationStandardOffset=0  TranslationStandardOffsetUnits=m  TranslationROffset=0  TranslationROffsetUnits=m  TranslationThetaOffset=0  TranslationThetaOffsetUnits=deg  TranslationZOffset=0  TranslationZOffsetUnits=m
  Rigid Transform3 : sm_lib/Frames and Transforms/Rigid Transform  RotationMethod=StandardAxis  FollAlignAxisA=+X  BaseAlignAxisA=+Y  FollAlignAxisB=+Y  BaseAlignAxisB=+Z  RotationStandardAxis=+X  RotationAngle=pi  RotationAngleUnits=rad  RotationArbitraryAxis=[0 0 1]  RotationSequenceAxes=FollowerAxes  RotationSequence=XYX  RotationSequenceAngles=[0 0 0]  RotationSequenceAnglesUnits=deg  RotationMatrix=[1 0 0; 0 1 0; 0 0 1]  Quaternion=[1 0 0 0]  TranslationMethod=None  TranslationCartesianOffset=[0 0 0]  TranslationCartesianOffsetUnits=m  TranslationStandardAxis=+X  TranslationStandardOffset=0  TranslationStandardOffsetUnits=m  TranslationROffset=0  TranslationROffsetUnits=m  TranslationThetaOffset=0  TranslationThetaOffsetUnits=deg  TranslationZOffset=0  TranslationZOffsetUnits=m
  Roll dof : Subsystem
  Simulink-PS Converter1 : nesl_utility_internal/Simulink-PS Converter  PhysicalDomain=network_engine_domain  SubClassName=ps_input  LeftPortType=input  RightPortType=output  PseudoPeriodic=off  Frequencies=[]  NoiseDistribution=none  NoiseParameters=[]  Unit=1  AffineConversion=off  FilteringAndDerivatives=provide  SimscapeFilterOrder=1  InputFilterTimeConstant=0.001  UdotUserProvided=0
  World Frame : sm_lib/Frames and Transforms/World Frame
  dofPitch : Subsystem
  Hub : PMIOPort  Side=Left
  CP : PMIOPort  Port=2  Side=Left
  omega : Outport
  omegadot : Outport  Port=2
  A,V,P_WhlRoll : Outport  Port=3
  Info_CP : Outport  Port=4
  wires:
  Bus Creator/1 -> Info_CP/1
  CPSensor/3(WhlCpZ) -> Bus Creator/3
  CPSensor/2(WhlCpY) -> Bus Creator/2
  CPSensor/1(WhlCpX) -> Bus Creator/1
  Roll dof/1(A,V,P_WhlRoll) -> A,V,P_WhlRoll/1
  Ext.F_T/1 -> Simulink-PS Converter1/1
  dofPitch/1(omega) -> omega/1  "omega"
  CPSensor/4(WhlCpVPsi) -> Bus Creator/4
  dofPitch/2(omegadot) -> omegadot/1
  connections:
  Simulink-PS Converter1/RConn1 -- External Force and Torque/LConn1
  External Force and Torque/RConn1 -- Rigid Transform2/LConn1 -- dofPitch/RConn1
  Cylindrical Solid/RConn1 -- Graphic/RConn1 -- Rigid Transform2/RConn1
  Pitch dof/LConn1 -- Hub/RConn1
  " Frame_CP"/RConn1 -- Roll dof/RConn1 -- Dummy mass/RConn1 -- CPSensor/RConn1 -- CP/RConn1 -- Angle Constraint/LConn1
  Rigid Transform1/RConn1 -- Roll dof/LConn1
  Rigid Transform3/LConn1 -- World Frame/RConn1
  Angle Constraint/RConn1 -- Rigid Transform3/RConn1
  dofPitch/LConn1 -- Rigid Transform1/LConn1 -- Pitch dof/RConn1

== system Out_of_Plane_Model/Chassis, Tires, and Areo/Chassis Body, Suspension, and Steering/CHASSIS/Steering and fork/Fork/fork (dofPrism)/fork/fork ==
  f : Inport
  Fork dof : sm_lib/Joints/Prismatic Joint  JointMode=Normal  CompositeWrenchDir=BaseOnFollower  CompositeWrenchFrame=BaseFrame  SenseConstraintForce=off  SenseConstraintTorque=off  SenseTotalForce=on  SenseTotalTorque=off  PositionTargetSpecify=on  PositionTargetPriority=High  PositionTargetValue=MotoFrntSuspEqlbrmLngth  PositionTargetValueUnits=m  VelocityTargetSpecify=on  VelocityTargetPriority=High  VelocityTargetValue=InitLwrFrkDerfmVel  VelocityTargetValueUnits=m/s  EquilibriumPosition=0  EquilibriumPositionUnits=m  SpringStiffness=0  SpringStiffnessUnits=N/m  DampingCoefficient=0  DampingCoefficientUnits=N/(m/s)  LowerLimitSpecify=off  LowerLimitBound=-1  LowerLimitBoundUnits=m  LowerLimitStiffness=1e6  LowerLimitStiffnessUnits=N/m  LowerLimitDamping=1e3  LowerLimitDampingUnits=N/(m/s)  LowerLimitTransitionRegionWidth=1e-4  LowerLimitTransitionRegionWidthUnits=m  UpperLimitSpecify=off  UpperLimitBound=1  UpperLimitBoundUnits=m  UpperLimitStiffness=1e6  UpperLimitStiffnessUnits=N/m  UpperLimitDamping=1e3  UpperLimitDampingUnits=N/(m/s)  UpperLimitTransitionRegionWidth=1e-4  UpperLimitTransitionRegionWidthUnits=m  TorqueActuationMode=InputTorque  MotionActuationMode=ComputedMotion  SensePosition=on  SenseVelocity=on  SenseAcceleration=on  SenseTorqueForce=off  SenseLowerLimitTorqueForce=off  SenseUpperLimitTorqueForce=off
  PS-Simulink Converter{1,4,8..9} (4 alike) : nesl_utility_internal/PS-Simulink Converter  PhysicalDomain=network_engine_domain  SubClassName=ps_output  LeftPortType=input  RightPortType=output  PseudoPeriodic=off  Frequencies=[]  VectorFormat=1-D array  Unit=inherit  AffineConversion=off
  Simulink-PS Converter : nesl_utility_internal/Simulink-PS Converter  PhysicalDomain=network_engine_domain  SubClassName=ps_input  LeftPortType=input  RightPortType=output  PseudoPeriodic=off  Frequencies=[]  NoiseDistribution=none  NoiseParameters=[]  Unit=1  AffineConversion=off  FilteringAndDerivatives=provide  SimscapeFilterOrder=1  InputFilterTimeConstant=0.001  UdotUserProvided=0
  B : PMIOPort  Side=Left
  F : PMIOPort  Port=2  Side=Right
  p : Outport
  v : Outport  Port=2
  a : Outport  Port=3
  ft : Outport  Port=4
  wires:
  f/1 -> Simulink-PS Converter/1
  PS-Simulink Converter4/1 -> p/1  "p"
  PS-Simulink Converter1/1 -> a/1
  PS-Simulink Converter8/1 -> v/1  "v"
  PS-Simulink Converter9/1 -> ft/1
  connections:
  Simulink-PS Converter/RConn1 -- Fork dof/LConn2
  Fork dof/LConn1 -- B/RConn1
  Fork dof/RConn2 -- PS-Simulink Converter4/LConn1
  Fork dof/RConn4 -- PS-Simulink Converter1/LConn1
  Fork dof/RConn5 -- PS-Simulink Converter9/LConn1
  Fork dof/RConn1 -- F/RConn1
  Fork dof/RConn3 -- PS-Simulink Converter8/LConn1

== system Out_of_Plane_Model/Chassis, Tires, and Areo/Chassis Body, Suspension, and Steering/CHASSIS/Steering and fork/Fork/fork (dofPrism)/fork/fork locked ==
  f : Inport
  Constant : Constant  Value=[0 0 0]
  Constant1 : Constant  Value=FrkFrL0
  Constant2 : Constant  Value=0
  Fork len : sm_lib/Frames and Transforms/Rigid Transform  RotationMethod=None  FollAlignAxisA=+X  BaseAlignAxisA=+Y  FollAlignAxisB=+Y  BaseAlignAxisB=+Z  RotationStandardAxis=+X  RotationAngle=0  RotationAngleUnits=rad  RotationArbitraryAxis=[0 0 1]  RotationSequenceAxes=FollowerAxes  RotationSequence=XYX  RotationSequenceAngles=[0 0 0]  RotationSequenceAnglesUnits=deg  RotationMatrix=[1 0 0; 0 1 0; 0 0 1]  Quaternion=[1 0 0 0]  TranslationMethod=Cartesian  TranslationCartesianOffset=[0 0 FrkFrL0]  TranslationCartesianOffsetUnits=m  TranslationStandardAxis=+Z  TranslationStandardOffset=0  TranslationStandardOffsetUnits=m  TranslationROffset=0  TranslationROffsetUnits=m  TranslationThetaOffset=0  TranslationThetaOffsetUnits=deg  TranslationZOffset=0  TranslationZOffsetUnits=m
  Terminator : Terminator
  B : PMIOPort  Side=Left
  F : PMIOPort  Port=2  Side=Right
  p : Outport
  v : Outport  Port=2
  a : Outport  Port=3
  ft : Outport  Port=4
  wires:
  f/1 -> Terminator/1
  Constant2/1 -> v/1, a/1
  Constant1/1 -> p/1
  Constant/1 -> ft/1
  connections:
  Fork len/LConn1 -- B/RConn1
  Fork len/RConn1 -- F/RConn1

== system Out_of_Plane_Model/Chassis, Tires, and Areo/Tire/Front Tire/Linear Front Simscape Tire/Brake model/MW Brake/Brakes/Disk Brake ==
  BrkPrs : Inport
  Omega : Inport  Port=2
  Disk Brake : autolibsharedcoupling/Rotational Brake  BrakeType=Disc  rotType=No inertia  extInfo=off  Iyy=1  br=1e-3  omegao=0  mu_static=BrkFrntStcFricCff  mu_kinetic=BrkFrntKinFricCff  disk_abore=BrkFrntBrkActrBore  Rm=BrkFrntBrkPadMeanRadius  num_pads=BrkFrntPadNum  drum_abore=BrkFrntBrkActrBore  drum_a=BrkFrntShoePinToDrumCntrDst  drum_c=BrkFrntShoePinToFrcAppDst  drum_r=BrkFrntIntrnRadius  drum_theta1=BrkFrntShoePinToPadStartAng  drum_theta2=BrkFrntShoePinToPadEndAng  brake_p_bpt=BrkFrntBrkActrPrsBpt  brake_n_bpt=BrkFrntWhlSpdBpt  f_brake_t=BrkFrntBrkTrqTbl  aMode=2
      settings: LibrarySourceBlock=vehdynlibbrake/Disc Brake
  MyBrk : Outport  VectorParamsAs1DForOutWhenUnconnected=off
  wires:
  BrkPrs/1 -> Disk Brake/1
  Omega/1 -> Disk Brake/2
  Disk Brake/1 -> MyBrk/1

== system Out_of_Plane_Model/Chassis, Tires, and Areo/Tire/Front Tire/Linear Front Simscape Tire/Brake model/MW Brake/Brakes/Drum Brake ==
  BrkPrs : Inport
  Omega : Inport  Port=2
  Drum Brake : autolibsharedcoupling/Rotational Brake  BrakeType=Drum  rotType=No inertia  extInfo=off  Iyy=1  br=1e-3  omegao=0  mu_static=BrkFrntStcFricCff  mu_kinetic=BrkFrntKinFricCff  disk_abore=BrkFrntBrkActrBore  Rm=BrkFrntBrkPadMeanRadius  num_pads=BrkFrntPadNum  drum_abore=BrkFrntBrkActrBore  drum_a=BrkFrntShoePinToDrumCntrDst  drum_c=BrkFrntShoePinToFrcAppDst  drum_r=BrkFrntIntrnRadius  drum_theta1=BrkFrntShoePinToPadStartAng  drum_theta2=BrkFrntShoePinToPadEndAng  brake_p_bpt=BrkFrntBrkActrPrsBpt  brake_n_bpt=BrkFrntWhlSpdBpt  f_brake_t=BrkFrntBrkTrqTbl  aMode=2
      settings: LibrarySourceBlock=vehdynlibbrake/Disc Brake
  MyBrk : Outport  VectorParamsAs1DForOutWhenUnconnected=off
  wires:
  Drum Brake/1 -> MyBrk/1
  Omega/1 -> Drum Brake/2
  BrkPrs/1 -> Drum Brake/1

== system Out_of_Plane_Model/Chassis, Tires, and Areo/Tire/Front Tire/Linear Front Simscape Tire/Brake model/MW Brake/Brakes/Mapped Brake ==
  BrkPrs : Inport
  Omega : Inport  Port=2
  Mapped Brake : autolibsharedcoupling/Rotational Brake  BrakeType=Mapped  rotType=No inertia  extInfo=off  Iyy=1  br=1e-3  omegao=0  mu_static=BrkFrntStcFricCff  mu_kinetic=BrkFrntKinFricCff  disk_abore=BrkFrntBrkActrBore  Rm=BrkFrntBrkPadMeanRadius  num_pads=BrkFrntPadNum  drum_abore=BrkFrntBrkActrBore  drum_a=BrkFrntShoePinToDrumCntrDst  drum_c=BrkFrntShoePinToFrcAppDst  drum_r=BrkFrntIntrnRadius  drum_theta1=BrkFrntShoePinToPadStartAng  drum_theta2=BrkFrntShoePinToPadEndAng  brake_p_bpt=BrkFrntBrkActrPrsBpt  brake_n_bpt=BrkFrntWhlSpdBpt  f_brake_t=BrkFrntBrkTrqTbl  aMode=2
      settings: LibrarySourceBlock=vehdynlibbrake/Disc Brake
  MyBrk : Outport  VectorParamsAs1DForOutWhenUnconnected=off
  wires:
  Omega/1 -> Mapped Brake/2
  Mapped Brake/1 -> MyBrk/1
  BrkPrs/1 -> Mapped Brake/1
